simulink model "A24"  (R2018b)
settings: Solver=FixedStepAuto  StartTime=0.0  StopTime=5.0  RelTol=1e-3  EnableMultiTasking=on
undefined symbols (not defined in the file): bound, clamping, k1, k2, minTorque, setValue, tau
libraries: simulink x2, arduinolib x1
settings Model: SimulationMode=external  ExtModeTrigDuration=2  Creator=bill  LastModifiedBy=bill
settings OptimizationCC: EnhancedBackFolding=on  PassReuseOutputArgsAs=Individual arguments  MaxStackSize=64  OptimizeBlockOrder=speed  DifferentSizesBufferReuse=on  OptimizationCustomize=off
settings DebuggingCC: ParameterTunabilityLossMsg=error
settings HardwareCC: ProdBitPerInt=16  ProdBitPerPointer=16  ProdBitPerSizeT=16  ProdBitPerPtrDiffT=16  ProdLargestAtomicFloat=None  ProdWordSize=8  ProdHWDeviceType=Atmel->AVR  UseEmbeddedCoderFeatures=off  UseSimulinkCoderFeatures=off
settings SFSimCC: MATLABDynamicMemAlloc=off
settings RTWCC: SystemTargetFile=ert.tlc  HardwareBoard=Arduino Uno  TemplateMakefile=ert_default_tmf  GenerateReport=on  Toolchain=Arduino AVR  BuildConfiguration=Faster Runs  IncludeHyperlinkInReport=on  LaunchReport=on  GenerateTraceInfo=on  GenerateTraceReport=on  GenerateTraceReportSl=on  GenerateTraceReportSf=on  GenerateTraceReportEml=on
settings CodeAppCC: ForceParamTrailComments=on  IgnoreCustomStorageClasses=off  OperatorAnnotations=on  SimulinkDataObjDesc=on  SFDataObjDesc=on  InsertBlockDesc=on
settings ERTTargetCC: SupportContinuousTime=on  SupportNonInlinedSFcns=on  SupportVariableSizeSignals=on

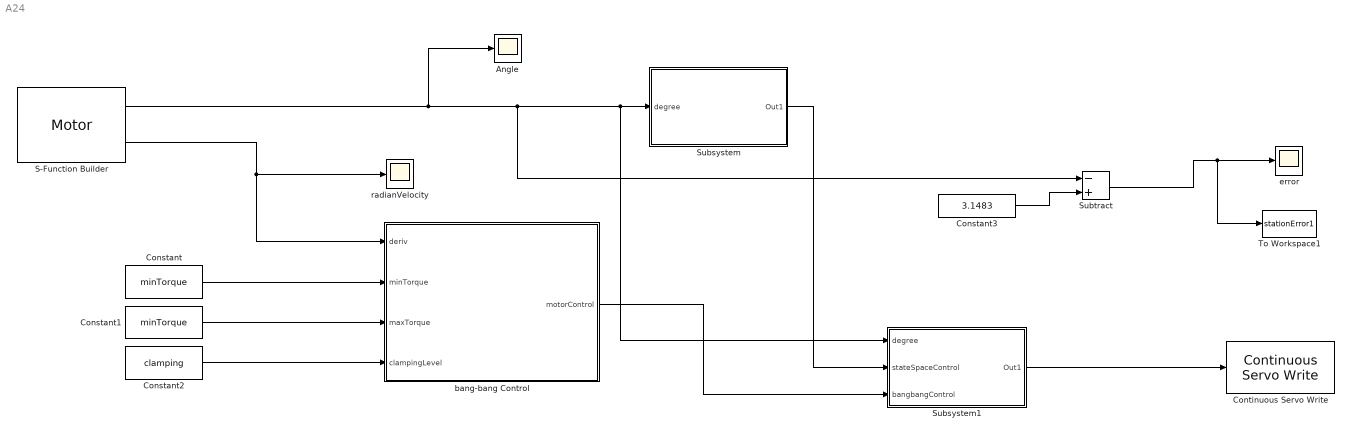
== system A24 ==
  Angle : Scope
  Constant : Constant  Value=minTorque
  Constant1 : Constant  Value=minTorque
  Constant2 : Constant  Value=clamping
  Constant3 : Constant  Value=3.1483
  Continuous Servo Write : arduinolib/Continuous Servo Write  pinNumber=7  ServoIndex=0  blockPlatform=ARDUINO
      settings: SourceProductName=Simulink Support Package for Arduino Hardware  SourceProductBaseCode=ARDUINO
  S-Function Builder : S-Function  InitFcn=try, set_param(gcb,'FunctionName','Motor'), end  FunctionName=Motor  SFunctionModules=Motor_wrapper  SFunctionDeploymentMode=off  EnableBusSupport=off  mask(S-Function Builder){}
      mask help: Simulink:masks:SFunctionBuilder_MD
      mask init:
      | val = [[.9  0.75 0.75 1 1 .9 .9 1]',[1 1 0.75 0.75 .9 .9 1 .9]'];try , sys = get_param(gcb,'SfunBuilderFcnName');if isempty(sys), sys = get_param(gcb,'FunctionName'); end,catch, sys = get_param(gcb,'FunctionName'); end
      settings: CopyFcn=set_param(gcbh,'LinkStatus','none')  PreSaveFcn=try, set_param(gcb,'FunctionName','Motor'), end  OpenFcn=sfunctionwizard(gcbh)
      mask Display: plot(val(:,1),val(:,2)),disp(sys), port_label('output',1,'posRad'), port_label('output',2,'deriv')
  Subsystem : Subsystem
  Subsystem1 : Subsystem
  Subtract : Sum  Inputs=-+
  To Workspace1 : ToWorkspace  VariableName=stationError1  SampleTime=-1
  bang-bang Control : MATLAB Function  TreatAsAtomicUnit=on
  error : Scope
  radianVelocity : Scope
  wires:
  S-Function Builder/2 -> radianVelocity/1, bang-bang Control/1(deriv)
  Constant/1 -> bang-bang Control/2(minTorque)
  Constant1/1 -> bang-bang Control/3(maxTorque)
  Constant2/1 -> bang-bang Control/4(clampingLevel)
  Subsystem1/1(Out1) -> Continuous Servo Write/1
  bang-bang Control/1(motorControl) -> Subsystem1/3(bangbangControl)
  Subsystem/1(Out1) -> Subsystem1/2("stateSpaceControl ")
  Subtract/1 -> To Workspace1/1, error/1
  S-Function Builder/1 -> Angle/1, Subtract/1, Subsystem1/1(degree), Subsystem/1(degree)
  Constant3/1 -> Subtract/2

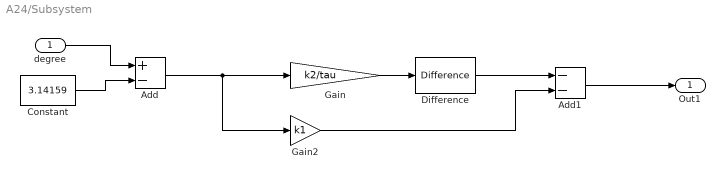
== system A24/Subsystem ==
  degree : Inport
  Add : Sum  Inputs=+-
  Add1 : Sum  Inputs=--
  Constant : Constant  Value=3.14159
  Difference : simulink/Discrete/Difference  ICPrevInput=0.0  OutMin=[]  OutMax=[]  OutDataType=fixdt(1, 16)  OutScaling=2^-10  DoSatur=off
  Gain : Gain  Gain=k2/tau
  Gain2 : Gain  Gain=k1
  Out1 : Outport
  wires:
  degree/1 -> Add/1
  Add1/1 -> Out1/1
  Difference/1 -> Add1/1
  Constant/1 -> Add/2
  Gain/1 -> Difference/1
  Add/1 -> Gain/1, Gain2/1
  Gain2/1 -> Add1/2

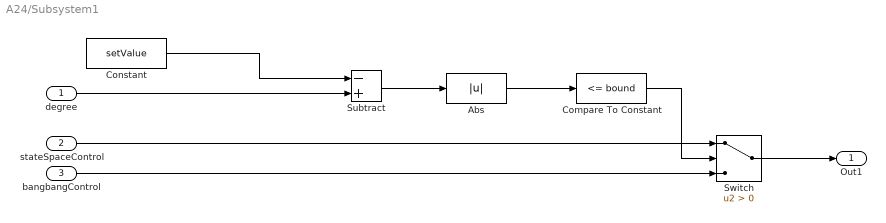
== system A24/Subsystem1 ==
  degree : Inport
  "stateSpaceControl " : Inport  Port=2
  bangbangControl : Inport  Port=3
  Abs : Abs
  Compare To Constant : simulink/Logic and Bit Operations/Compare To Constant  relop=<=  const=bound  OutDataTypeStr=boolean
  Constant : Constant  Value=setValue
  Subtract : Sum  Inputs=-+
  Switch : Switch  Criteria=u2 > Threshold
  Out1 : Outport
  wires:
  degree/1 -> Subtract/2
  Constant/1 -> Subtract/1
  Subtract/1 -> Abs/1
  Abs/1 -> Compare To Constant/1
  "stateSpaceControl "/1 -> Switch/1
  bangbangControl/1 -> Switch/3
  Compare To Constant/1 -> Switch/2
  Switch/1 -> Out1/1

== matlab function A24/bang-bang Control ==
  data: deriv input; motorControl output; minTorque input; maxTorque input; clampingLevel input
function motorControl  = fcn(deriv,minTorque, maxTorque, clampingLevel)
    persistent  drive lastDeriv signDeriv clamping;
    if(isempty(drive))
        drive = int16(15);
        lastDeriv = 0;
        signDeriv = 0;
        clamping = 0;
    end

    if(deriv==0)
        if(~clamping)
            if(lastDeriv > 0)
                drive = int16(maxTorque);
            else
                drive = int16(minTorque);
            end
            clamping = 1;
            signDeriv = lastDeriv;
        end
    end
    
    if(clamping)
        if(signDeriv > 0 && deriv < (-1 * clampingLevel))
            clamping  = 0;
        elseif(signDeriv < 0 && deriv > clampingLevel)
            clamping = 0;
        end
    end
    
    lastDeriv = deriv;
    motorControl = double(drive);
